simulink model "noise_alias"  (Simulink 7.7)
settings: Solver=ode45  StartTime=0.0  StopTime=2  RelTol=1e-3
values from neighbouring files (symbols this model uses):
  frausch = 250    [analog_bp3.m]    (also in analog_tp2.m = 500)
  fs = 16000    [G722_1.m]    (also in TP_fdesign1.m = 0.215; adaptiv_2.m = 1000; adaptiv_3.m = 1000; adaptiv_4.m = 1000)
undefined symbols (not defined in the file or in its folder): fpsd, get
libraries: dsparch4 x2, dspspect3 x2, dspstat3 x2, dspsigops x2, dspsnks4 x1
settings Model: Creator=svenhoffmann  LastModifiedBy=josef  ExtModeAutoUpdateStatusClock=off
settings DataIOCC: MaxDataPoints=1  SignalLoggingName=sigsOut
settings DebuggingCC: SaveWithParameterizedLinksMsg=none  SignalResolutionControl=TryResolveAllWithWarning  SolverPrmCheckMsg=none  MultiTaskDSMMsg=warning  MultiTaskCondExecSysMsg=none  StrictBusMsg=None
settings HardwareCC: TargetUnknown=on
settings RTWCC: IncludeERTFirstTime=on

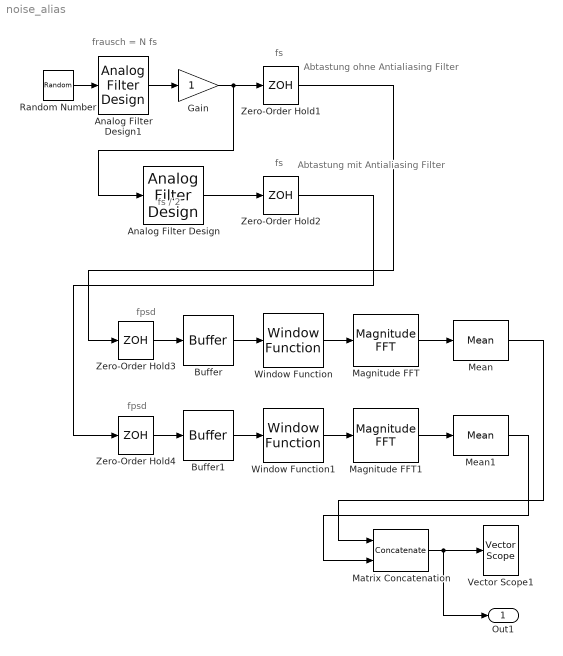
== system noise_alias ==
  note: frausch = N fs
  note: fs
  note: fs
  note: fs / 2
  note: fpsd
  note: fpsd
  note: Abtastung ohne Antialiasing
      | Filter
  note: Abtastung mit Antialiasing
      | Filter
  Analog Filter Design : dsparch4/Analog Filter Design  method=Butterworth  filttype=Lowpass  N=8  Wlo=2*pi*fs/2  Whi=80  Rp=2  Rs=40
  Analog Filter Design1 : dsparch4/Analog Filter Design  method=Butterworth  filttype=Lowpass  N=8  Wlo=2*pi*frausch  Whi=80  Rp=2  Rs=40
  Buffer : Buffer  N=256  V=64
  Buffer1 : Buffer  N=256  V=64
  Gain : Gain  SaturateOnIntegerOverflow=on  OutDataTypeStr=Inherit: Same as input  ParamDataTypeStr=Inherit: Same as input
  Magnitude FFT : dspspect3/Magnitude FFT  SystemSampleTime=-1  mag_or_magsq=Magnitude squared  fftLenInherit=off  fftsize=256
  Magnitude FFT1 : dspspect3/Magnitude FFT  SystemSampleTime=-1  mag_or_magsq=Magnitude squared  fftLenInherit=off  fftsize=256
  Matrix Concatenation : Concatenate  Mode=Multidimensional array  ConcatenateDimension=2
  Mean : dspstat3/Mean  run=on  reset_popup=None  InputProcessing=Inherited (this choice will be removed - see release notes)  directionMode=Each column  dimension=1  treatSBRowAsCol=on  roiEnable=off  roiType=Rectangles  roiPortion=Entire ROI  roiOutput=Individual statistics for each ROI  roiFlag=off  outputDataTypeStr=Inherit: Same as accumulator  outputLastDataTypeStr=Inherit: Same as accumulator  outputMin=[]  outputMax=[]  roundingMode=Floor  overflowMode=off
  Mean1 : dspstat3/Mean  run=on  reset_popup=None  InputProcessing=Inherited (this choice will be removed - see release notes)  directionMode=Each column  dimension=1  treatSBRowAsCol=on  roiEnable=off  roiType=Rectangles  roiPortion=Entire ROI  roiOutput=Individual statistics for each ROI  roiFlag=off  outputDataTypeStr=Inherit: Same as accumulator  outputLastDataTypeStr=Inherit: Same as accumulator  outputMin=[]  outputMax=[]  roundingMode=Floor  overflowMode=off
  Random Number : RandomNumber  SampleTime=0
  Vector Scope1 : dspsnks4/Vector Scope  ScopeProperties=off  Domain=Frequency  HorizSpan=1  DisplayProperties=off  AxisGrid=on  Memory=off  FrameNumber=on  AxisLegend=off  AxisZoom=off  OpenScopeAtSimStart=on  OpenScopeImmediately=off  FigPos=get(0,'defaultfigureposition')  AxisProperties=on  XUnits=Hertz  XRange=[0...Fs/2]  InheritXIncr=off  XIncr=1/6000  XLabel=Time  XLimit=Auto  XMin=0  XMax=1  XStart=0  YUnits=dB  YLabel=Amplitude  LineProperties=off  XAxisParamsVer=6.8
      settings: YMin=-31.8349324142458  YMax=20.5995421669601
  Window Function : dspsigops/Window Function  winmode=Apply window to input  wintype=Hamming  sampmode=Continuous  samptime=1  N=64  Rs=50  beta=10  winsamp=Symmetric  UserWindow=hamming  OptParams=off  UserParams={1.0}  RowConvenienceOn=on  dataType=double  isSigned=on  wordLen=16  udDataType=sfix(16)  fracBitsMode=Best precision  numFracBits=15  roundingMode=Floor  overflowMode=off  numSidelobes=4  sidelobeLevel=-30
  Window Function1 : dspsigops/Window Function  winmode=Apply window to input  wintype=Hamming  sampmode=Continuous  samptime=1  N=64  Rs=50  beta=10  winsamp=Symmetric  UserWindow=hamming  OptParams=off  UserParams={1.0}  RowConvenienceOn=on  dataType=double  isSigned=on  wordLen=16  udDataType=sfix(16)  fracBitsMode=Best precision  numFracBits=15  roundingMode=Floor  overflowMode=off  numSidelobes=4  sidelobeLevel=-30
  Zero-Order Hold1 : ZeroOrderHold  SampleTime=1/fs
  Zero-Order Hold2 : ZeroOrderHold  SampleTime=1/fs
  Zero-Order Hold3 : ZeroOrderHold  SampleTime=1/fpsd
  Zero-Order Hold4 : ZeroOrderHold  SampleTime=1/fpsd
  Out1 : Outport
  wires:
  Random Number/1 -> Analog Filter Design1/1
  Analog Filter Design1/1 -> Gain/1
  Buffer/1 -> Window Function/1
  Buffer1/1 -> Window Function1/1
  Analog Filter Design/1 -> Zero-Order Hold2/1
  Magnitude FFT/1 -> Mean/1
  Magnitude FFT1/1 -> Mean1/1
  Matrix Concatenation/1 -> Out1/1, Vector Scope1/1
  Gain/1 -> Zero-Order Hold1/1, Analog Filter Design/1
  Zero-Order Hold3/1 -> Buffer/1
  Zero-Order Hold4/1 -> Buffer1/1
  Window Function/1 -> Magnitude FFT/1
  Window Function1/1 -> Magnitude FFT1/1
  Zero-Order Hold1/1 -> Zero-Order Hold3/1
  Zero-Order Hold2/1 -> Zero-Order Hold4/1
  Mean/1 -> Matrix Concatenation/1
  Mean1/1 -> Matrix Concatenation/2
